simulink model "State_controller_real_stabilized"  (Simulink 7.9)
settings: Solver=ode3  StartTime=0.0  StopTime=100  RelTol=1e-3
undefined symbols (not defined in the file or in its folder): sigbuilder_block
libraries: simulink x1
settings Model: Creator=dAN  LastModifiedBy=dAN

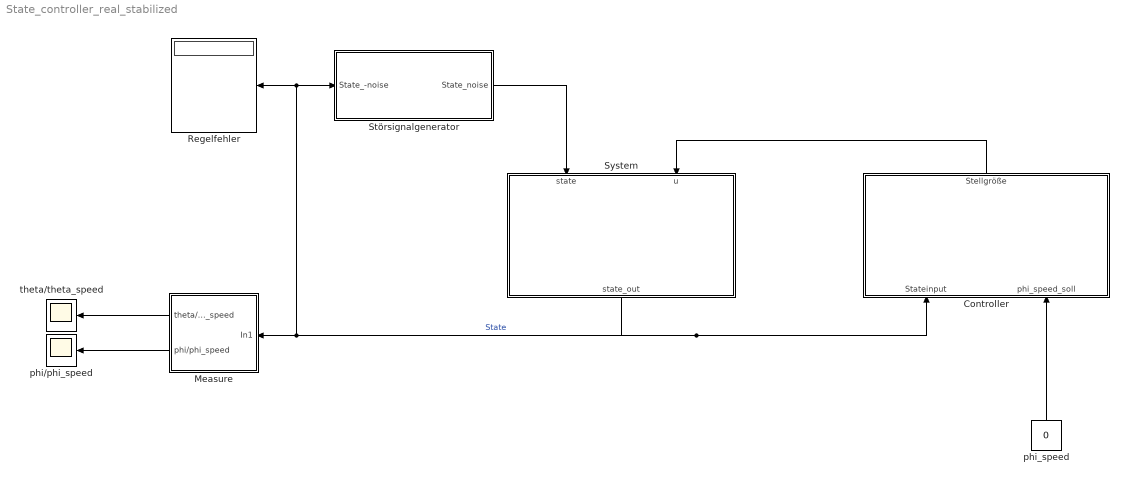
== system State_controller_real_stabilized ==
  Controller : Subsystem
  Measure : Subsystem
  Regelfehler : Display
  Störsignalgenerator : Subsystem
  System : Subsystem
  phi/phi_speed : Scope
  phi_speed : Constant  Value=0
  theta/theta_speed : Scope
  wires:
  Controller/1(Stellgröße) -> System/2(u)
  Störsignalgenerator/1(State_noise) -> System/1(state)
  phi_speed/1 -> Controller/2(phi_speed_soll)
  System/1(state_out) -> Controller/1(Stateinput), Measure/1(In1), Störsignalgenerator/1(State_-noise), Regelfehler/1  "State"
  Measure/2(phi/phi_speed) -> phi/phi_speed/1
  Measure/1(theta/theta_speed) -> theta/theta_speed/1

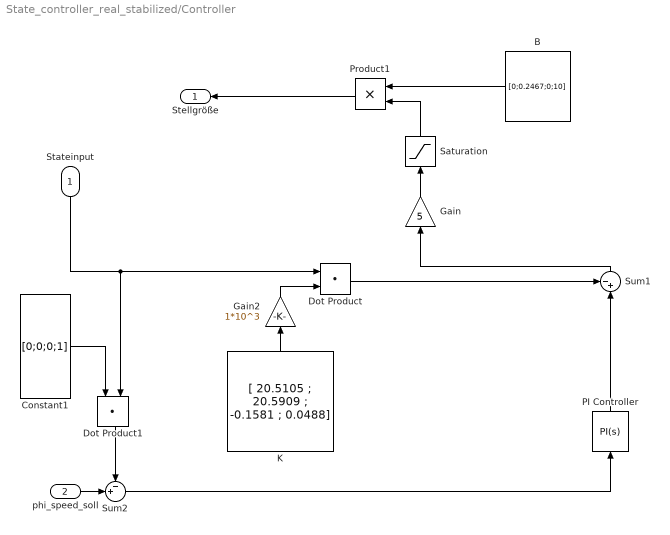
== system State_controller_real_stabilized/Controller ==
  Stateinput : Inport
  phi_speed_soll : Inport  Port=2
  B : Constant  Value=[0;0.2467;0;10]  VectorParams1D=off
  Constant1 : Constant  Value=[0;0;0;1]  VectorParams1D=off
  Dot Product : DotProduct  InputSameDT=on  OutDataTypeStr=Inherit: Inherit via internal rule
  Dot Product1 : DotProduct  InputSameDT=on  OutDataTypeStr=Inherit: Inherit via internal rule
  Gain : Gain  Gain=5
  Gain2 : Gain  Gain=1*10^3
  K : Constant  Value="[ 20.5105 ;  20.5909 ;  -0.1581 ;   0.0488]"  VectorParams1D=off
  PI Controller : simulink/Continuous/PID Controller  Controller=PI  TimeDomain=Continuous-time  SampleTime=1  IntegratorMethod=Forward Euler  FilterMethod=Forward Euler  Form=Parallel  P=1  I=5  D=0  N=100  InitialConditionSource=internal  InitialConditionForIntegrator=0  InitialConditionForFilter=0  ExternalReset=none  LimitOutput=off  UpperSaturationLimit=inf  LowerSaturationLimit=-inf  LinearizeAsGain=off  AntiWindupMode=none  Kb=1  TrackingMode=off  Kt=1  PParamMin=[]  PParamMax=[]  IParamMin=[]  IParamMax=[]  DParamMin=[]  DParamMax=[]  NParamMin=[]  NParamMax=[]  KbParamMin=[]  KbParamMax=[]  KtParamMin=[]  KtParamMax=[]  POutMin=[]  POutMax=[]  IOutMin=[]  IOutMax=[]  DOutMin=[]  DOutMax=[]  NOutMin=[]  NOutMax=[]  KbOutMin=[]  KbOutMax=[]  KtOutMin=[]  KtOutMax=[]  IntegratorOutMin=[]  IntegratorOutMax=[]  FilterOutMin=[]  FilterOutMax=[]  SumOutMin=[]  SumOutMax=[]  SumI1OutMin=[]  SumI1OutMax=[]  SumI2OutMin=[]  SumI2OutMax=[]  SumI3OutMin=[]  SumI3OutMax=[]  SumDOutMin=[]  SumDOutMax=[]  SaturationOutMin=[]  SaturationOutMax=[]  IntegratorContinuousStateAttributes=''  IntegratorStateMustResolveToSignalObject=off  IntegratorRTWStateStorageClass=Auto  FilterContinuousStateAttributes=''  FilterStateMustResolveToSignalObject=off  FilterRTWStateStorageClass=Auto
  Product1 : Product  RndMeth=Zero
  Saturation : Saturate  UpperLimit=180  LowerLimit=-180
  Sum1 : Sum  Inputs=-+|
  Sum2 : Sum  Inputs=-+|
  Stellgröße : Outport
  wires:
  K/1 -> Gain2/1
  B/1 -> Product1/1
  Dot Product/1 -> Sum1/1
  Sum1/1 -> Gain/1
  Sum2/1 -> PI Controller/1
  Gain/1 -> Saturation/1
  Dot Product1/1 -> Sum2/1
  Gain2/1 -> Dot Product/2
  Constant1/1 -> Dot Product1/1
  PI Controller/1 -> Sum1/2
  Saturation/1 -> Product1/2
  Product1/1 -> Stellgröße/1
  Stateinput/1 -> Dot Product/1, Dot Product1/2
  phi_speed_soll/1 -> Sum2/2

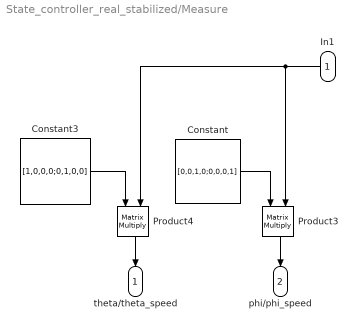
== system State_controller_real_stabilized/Measure ==
  In1 : Inport
  Constant : Constant  Value=[0,0,1,0;0,0,0,1]  VectorParams1D=off
  Constant3 : Constant  Value=[1,0,0,0;0,1,0,0]  VectorParams1D=off
  Product3 : Product  Multiplication=Matrix(*)  RndMeth=Zero
  Product4 : Product  Multiplication=Matrix(*)  RndMeth=Zero
  theta/theta_speed : Outport
  phi/phi_speed : Outport  Port=2
  wires:
  Constant/1 -> Product3/1
  Constant3/1 -> Product4/1
  In1/1 -> Product3/2, Product4/2
  Product4/1 -> theta/theta_speed/1
  Product3/1 -> phi/phi_speed/1

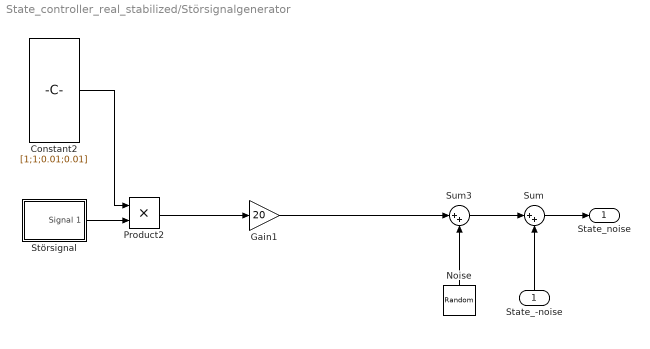
== system State_controller_real_stabilized/Störsignalgenerator ==
  State_-noise : Inport
  Constant2 : Constant  Value=[1;1;0.01;0.01]  VectorParams1D=off
  Gain1 : Gain  Gain=20
  Noise : UniformRandomNumber  Minimum=-[5;3;1;1]  Maximum=[5;3;1;1]  SampleTime=0.1  VectorParams1D=off
  Product2 : Product  RndMeth=Zero
  Störsignal : Subsystem  Tag=STV Subsys  LoadFcn=sigbuilder_block('load');  StartFcn=sigbuilder_block('start');  StopFcn=sigbuilder_block('stop');  ClipboardFcn=sigbuilder_block('clipboard');  mask(Sigbuilder block){}
      mask help: Simulink:masks:SigbuilderBlock_MD
      mask init:
      | if ~strcmp(get_param(bdroot(gcbh),'SimulationStatus'),'stopped') tuvar = sigbuilder_block('maskInit'); end
      settings: CopyFcn=sigbuilder_block('copy');  DeleteFcn=sigbuilder_block('delete');  ModelCloseFcn=sigbuilder_block('modelClose');  PreSaveFcn=sigbuilder_block('preSave');  PauseFcn=sigbuilder_block('pause');  ContinueFcn=sigbuilder_block('continue');  NameChangeFcn=sigbuilder_block('namechange');  OpenFcn=sigbuilder_block('open',[437.25 199.5 550.5 399.75 ]);  CloseFcn=sigbuilder_block('close');
      mask Display: plot(0, 0, 100, 100,[2, 2, 32, 32, 2], [68, 8, 8, 68, 68],[32, 2], [38, 38], [32, 19, 2],[53, 60, 44], [32, 17, 17, 2],[16, 16, 31, 31]);txt = getActiveGroup(gcbh);text(2, 100, txt,'verticalAlignment', 'top');
  Sum : Sum  Inputs=|++
  Sum3 : Sum  Inputs=|++
  State_noise : Outport
  wires:
  Product2/1 -> Gain1/1
  Constant2/1 -> Product2/1
  Störsignal/1(Signal 1) -> Product2/2
  Noise/1 -> Sum3/2
  Sum3/1 -> Sum/1
  State_-noise/1 -> Sum/2
  Sum/1 -> State_noise/1
  Gain1/1 -> Sum3/1

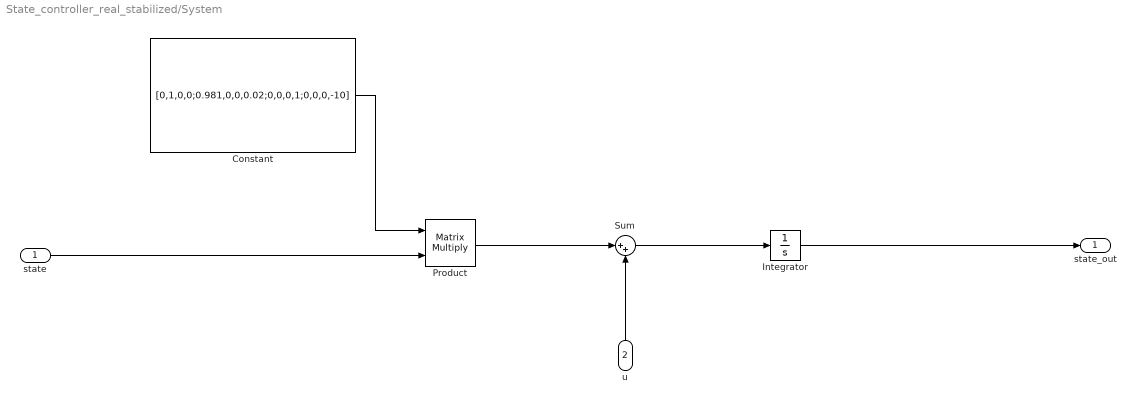
== system State_controller_real_stabilized/System ==
  state : Inport
  u : Inport  Port=2
  Constant : Constant  Value=[0,1,0,0;0.981,0,0,0.02;0,0,0,1;0,0,0,-10]  VectorParams1D=off
  Integrator : Integrator
  Product : Product  Multiplication=Matrix(*)  RndMeth=Zero
  Sum : Sum  Inputs=|++
  state_out : Outport
  wires:
  Integrator/1 -> state_out/1
  Constant/1 -> Product/1
  state/1 -> Product/2
  Sum/1 -> Integrator/1
  u/1 -> Sum/2
  Product/1 -> Sum/1

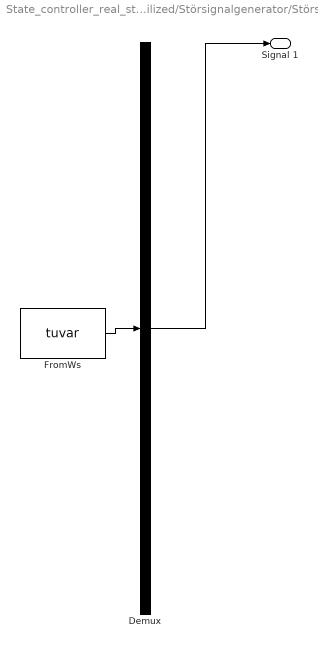
== system State_controller_real_stabilized/Störsignalgenerator/Störsignal ==
  Demux : Demux  Tag=STV Demux  Outputs=1
  FromWs : FromWorkspace  Tag=STV FromWs  VariableName=tuvar  SampleTime=0  SigBuilderData=DataTag0  VnvData=DataTag1
      SigBuilderData=|
      | common.afterFinalStr = 'Extrapolate'
      | common.sampleTime = 0
      | dataSet.timeRange = [0 10]
      | dataSet.name = 'Group 1'
      | sbobj.Groups.Name = 'Group 1'
      | sbobj.Groups.Signals.Name = 'Signal 1'
      | sbobj.Groups.Signals.XData = [0 1.02 1.02 2 2 10]
      | sbobj.Groups.Signals.YData = [0.005 0.005 1 1 0.005 0.005]
  Signal 1 : Outport  Tag=STV Outport
  wires:
  Demux/1 -> Signal 1/1
  FromWs/1 -> Demux/1
